simulink model "dstar_cpp_test"  (R2018a)
settings: Solver=VariableStepAuto  StartTime=0.0  StopTime=10.0  RelTol=1e-3
settings Model: Creator=alex  LastModifiedBy=alex

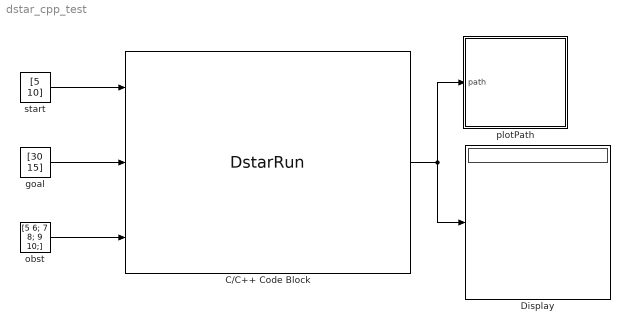
== system dstar_cpp_test ==
  C/C++ Code Block : S-Function  InitFcn=try, set_param(gcb,'FunctionName','DstarRun'), end  FunctionName=DstarRun  SFunctionModules=DstarRun_wrapper Dstar  SFunctionDeploymentMode=off  EnableBusSupport=off  mask(S-Function Builder){}
      mask help: Simulink:masks:SFunctionBuilder_MD
      mask init:
      | val = [[.9  0.75 0.75 1 1 .9 .9 1]',[1 1 0.75 0.75 .9 .9 1 .9]'];try , sys = get_param(gcb,'SfunBuilderFcnName');if isempty(sys), sys = get_param(gcb,'FunctionName'); end,catch, sys = get_param(gcb,'FunctionName'); end
      settings: CopyFcn=set_param(gcbh,'LinkStatus','none')  PreSaveFcn=try, set_param(gcb,'FunctionName','DstarRun'), end  OpenFcn=sfunctionwizard(gcbh)
      mask Display: plot(val(:,1),val(:,2)),disp(sys), port_label('input',1,'start'), port_label('input',2,'goal'), port_label('input',3,'obst'), port_label('output',1,'shortPath')
  Display : Display
  goal : Constant  Value=[30 15]
  "obst " : Constant  Value=[5 6; 7 8; 9 10;]  VectorParams1D=off
  "plotPath " : MATLAB Function  TreatAsAtomicUnit=on
  "start " : Constant  Value=[5 10]
  wires:
  "start "/1 -> C/C++ Code Block/1
  goal/1 -> C/C++ Code Block/2
  C/C++ Code Block/1 -> "plotPath "/1(path), Display/1
  "obst "/1 -> C/C++ Code Block/3

== matlab function dstar_cpp_test/plotPath  ==
  data: path input
function plotPath(path)
plot(path(:,1),path(:,2), 'b*');
xlim([0 60]);
ylim([0 40]);
end
